simulink library "myLibrary"  (R2024b)
settings: Solver=VariableStepAuto  StartTime=0.0  StopTime=10.0  RelTol=1e-3
values from neighbouring files (symbols this model uses):
  Ts = 2.222222e-4    (= 0.0002222222)    [Lowpass.m]
undefined symbols (not defined in the file or in its folder): Ki, Kp
settings Model: Creator=SESA504213  LastModifiedBy=SESA504213

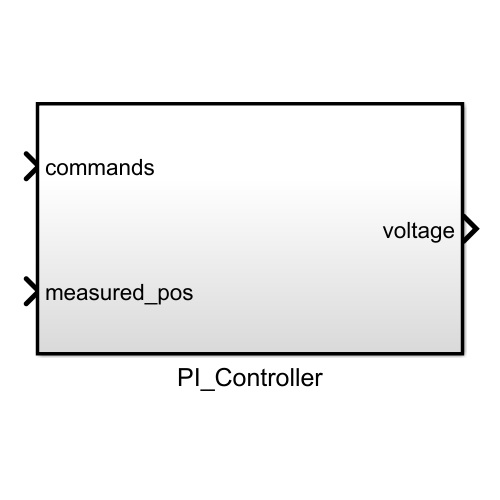
[thumbnail: Simulink's stored preview of the top-level diagram]
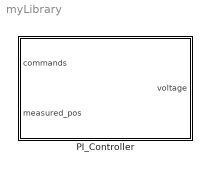
== system myLibrary ==
  PI_Controller : Subsystem  TreatAsAtomicUnit=on

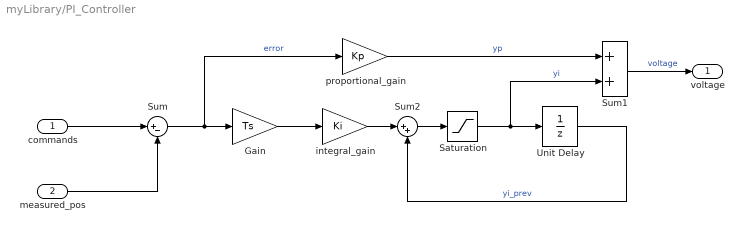
== system myLibrary/PI_Controller ==
  commands : Inport
  measured_pos : Inport  Port=2
  Gain : Gain  Gain=Ts  SaturateOnIntegerOverflow=on  OutDataTypeStr=Inherit: Same as input  ParamDataTypeStr=Inherit: Same as input
  Saturation : Saturate  UpperLimit=12  LowerLimit=-12
  Sum : Sum  Inputs=|+-
  Sum1 : Sum  InputSameDT=on  SaturateOnIntegerOverflow=on  OutDataTypeStr=Inherit: Same as first input
  Sum2 : Sum  Inputs=|++  InputSameDT=on  SaturateOnIntegerOverflow=on  OutDataTypeStr=Inherit: Same as first input
  Unit Delay : UnitDelay  SampleTime=Ts  HasFrameUpgradeWarning=on
  integral_gain : Gain  Gain=Ki  SaturateOnIntegerOverflow=on  OutDataTypeStr=Inherit: Same as input  ParamDataTypeStr=Inherit: Same as input
  proportional_gain : Gain  Gain=Kp  SaturateOnIntegerOverflow=on  OutDataTypeStr=Inherit: Same as input  ParamDataTypeStr=Inherit: Same as input
  voltage : Outport
  wires:
  proportional_gain/1 -> Sum1/1  "yp"
  Sum1/1 -> voltage/1  "voltage"
  Unit Delay/1 -> Sum2/2  "yi_prev"
  integral_gain/1 -> Sum2/1
  Gain/1 -> integral_gain/1
  Saturation/1 -> Sum1/2, Unit Delay/1  "yi"
  Sum2/1 -> Saturation/1
  commands/1 -> Sum/1
  Sum/1 -> Gain/1, proportional_gain/1  "error"
  measured_pos/1 -> Sum/2
